simulink model "Coder_8_4"  (R2017a)
settings: Solver=ode45  StartTime=0.0  StopTime=1e-3  RelTol=1e-3  EnableMultiTasking=on
settings Model: Creator=robertoeduardo  LastModifiedBy=Jesus
settings DataIOCC: LimitDataPoints=on  SaveFormat=Array
settings OptimizationCC: LifeSpan=inf
settings DebuggingCC: UnderspecifiedInitializationDetection=Classic  MergeDetectMultiDrivingBlocksExec=none  SolverPrmCheckMsg=warning  SFUnexpectedBacktrackingDiag=warning  SFNoUnconditionalDefaultTransitionDiag=warning  SFExecutionAtInitializationDiag=none
settings HardwareCC: ProdBitPerPointer=32  ProdBitPerSizeT=32  ProdBitPerPtrDiffT=32  ProdLargestAtomicFloat=None  ProdIntDivRoundTo=Undefined  ProdEndianess=Unspecified  ProdWordSize=32  ProdHWDeviceType=32-bit Generic
settings ModelReferenceCC: PropagateSignalLabelsOutOfModel=off
settings GRTTargetCC: TargetLangStandard=C89/C90 (ANSI)  GeneratePreprocessorConditionals=Disable all
settings ConfigComp: CovMetricSettings=dw  CovHtmlReporting=on  CovSaveCumulativeToWorkspaceVar=on  CovSaveSingleToWorkspaceVar=on  CovExternalEMLEnable=off

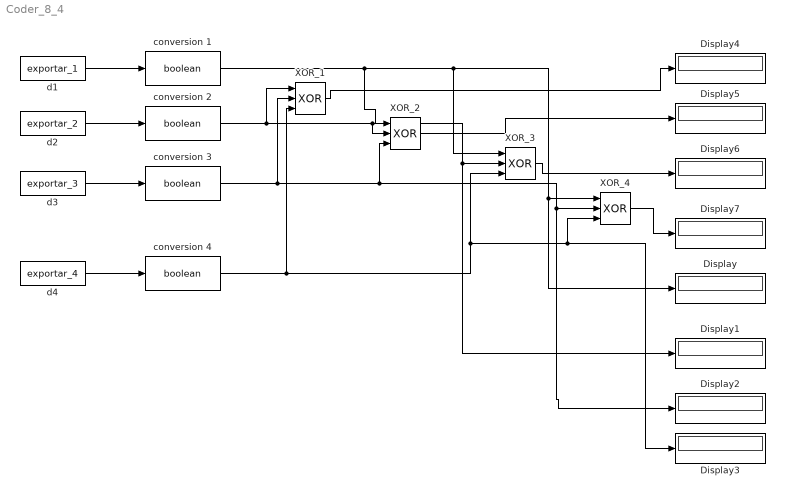
== system Coder_8_4 ==
  Display{,1..7} (8 alike) : Display
  XOR_{1..4} (4 alike) : Logic  Operator=XOR  Inputs=3  IconShape=distinctive  AllPortsSameDT=off  OutDataTypeStr=boolean
  conversion {1..4} (4 alike) : DataTypeConversion  OutDataTypeStr=boolean
  d1 : FromWorkspace  VariableName=exportar_1  SampleTime=0
  d2 : FromWorkspace  VariableName=exportar_2  SampleTime=0
  d3 : FromWorkspace  VariableName=exportar_3  SampleTime=0
  d4 : FromWorkspace  VariableName=exportar_4  SampleTime=0
  wires:
  d1/1 -> conversion 1/1
  d2/1 -> conversion 2/1
  d3/1 -> conversion 3/1
  d4/1 -> conversion 4/1
  conversion 2/1 -> XOR_2/2, Display1/1, XOR_3/2, XOR_1/1
  conversion 3/1 -> XOR_2/3, Display2/1, XOR_4/2, XOR_1/2
  conversion 4/1 -> XOR_1/3, XOR_3/3, XOR_4/3, Display3/1
  conversion 1/1 -> XOR_3/1, Display/1, XOR_4/1, XOR_2/1
  XOR_1/1 -> Display4/1
  XOR_2/1 -> Display5/1
  XOR_3/1 -> Display6/1
  XOR_4/1 -> Display7/1
